simulink model "dsPIC33CK_Curiosity_CRL_ExternalMode"  (R2020b)
settings: Solver=FixedStepDiscrete  StartTime=0.0  StopTime=inf  FixedStep=0.01  RelTol=1e-3
undefined symbols (not defined in the file): B0, D3, D4, Max, MaxPer, ms, P32, P67, P68, Pin, Resol, Timer, us
libraries: MCHP_Blockset x9
(part 1 of 2)
settings Model: SimulationMode=external  ExtModeTrigDuration=1  Creator=M17129  LastModifiedBy=Lubin Kerhuel
settings DataIOCC: ReturnWorkspaceOutputs=off
settings OptimizationCC: DefaultUnderspecifiedDataType=single  EfficientTunableParamExpr=on
settings DebuggingCC: ParameterTunabilityLossMsg=error  ArithmeticOperatorsInVariantConditions=warning
settings HardwareCC: ProdBitPerInt=16  ProdBitPerPointer=16  ProdBitPerSizeT=16  ProdBitPerPtrDiffT=16  ProdLargestAtomicInteger=Integer  ProdLargestAtomicFloat=None  ProdWordSize=16  ProdHWDeviceType=Generic->Custom
settings ModelReferenceCC: ModelReferenceNumInstancesAllowed=Single
settings SFSimCC: SimUseLocalCustomCode=off  MATLABDynamicMemAlloc=off  CustomCodeUndefinedFunction=UseInterfaceOnly
settings RTWCC: Description=Microchip Embedded Target PIC24 dsPIC30 dsPIC33 (real-time)  SystemTargetFile=MCHP_dsPIC_stf.tlc  TemplateMakefile=MCHP_dsPIC.tmf  GenerateReport=on  RTWUseLocalCustomCode=off  IncludeHyperlinkInReport=on  LaunchReport=on  CodeProfilingSaveOptions=AllData  GenerateTraceInfo=on  GenerateTraceReport=on  GenerateTraceReportSl=on  GenerateTraceReportSf=on  GenerateTraceReportEml=on  GenerateWebview=on  GenerateCodeMetricsReport=on  GenerateCodeReplacementReport=on
settings CodeAppCC: ForceParamTrailComments=on  IgnoreCustomStorageClasses=off  MaxIdLength=255  OperatorAnnotations=on  SimulinkDataObjDesc=on  SFDataObjDesc=on  InsertBlockDesc=on
settings STFCustomTargetCC: TargetLibSuffix=_lib.a  CodeReplacementLibrary=Microchip Code Replacement Library for dsPIC  MultiwordLength=256  ConcurrentExecutionCompliant=off  IncludeMdlTerminateFcn=off  CombineOutputUpdateFcns=on  CombineSignalStateStructs=on  ERTCustomFileBanners=on  SupportContinuousTime=off  RemoveResetFunc=on  MATLABClassNameForMDSCustomization=Simulink.SoftwareTarget.ERTCustomization  CPPClassGenCompliant=off  GRTInterface=off  SystemTargetFile=MCHP_dsPIC_stf.tlc
settings ERTTargetCC: TargetLibSuffix=_lib.a  CodeReplacementLibrary=Microchip Code Replacement Library for dsPIC  ParMdlRefBuildCompliant=off  CompOptLevelCompliant=off  ConcurrentExecutionCompliant=off  IncludeMdlTerminateFcn=off  CombineSignalStateStructs=on  SupportNonInlinedSFcns=on  ModelStepFunctionPrototypeControlCompliant=off  CPPClassGenCompliant=off  UseToolchainInfoCompliant=off  ExtMode=on  ExtModeTransport=1  ExtModeStaticAllocSize=1024  ExtModeMexFile=ext_serial_win32_comm_no_acks  ExtModeMexArgs=1 10 460800  ERTSrcFileBannerTemplate=MCHP_dsPIC_code_template.cgt  ERTHdrFileBannerTemplate=MCHP_dsPIC_code_template.cgt  ERTDataSrcFileTemplate=MCHP_dsPIC_code_template.cgt  ERTDataHdrFileTemplate=MCHP_dsPIC_code_template.cgt  ERTCustomFileTemplate=MCHP_main.tlc

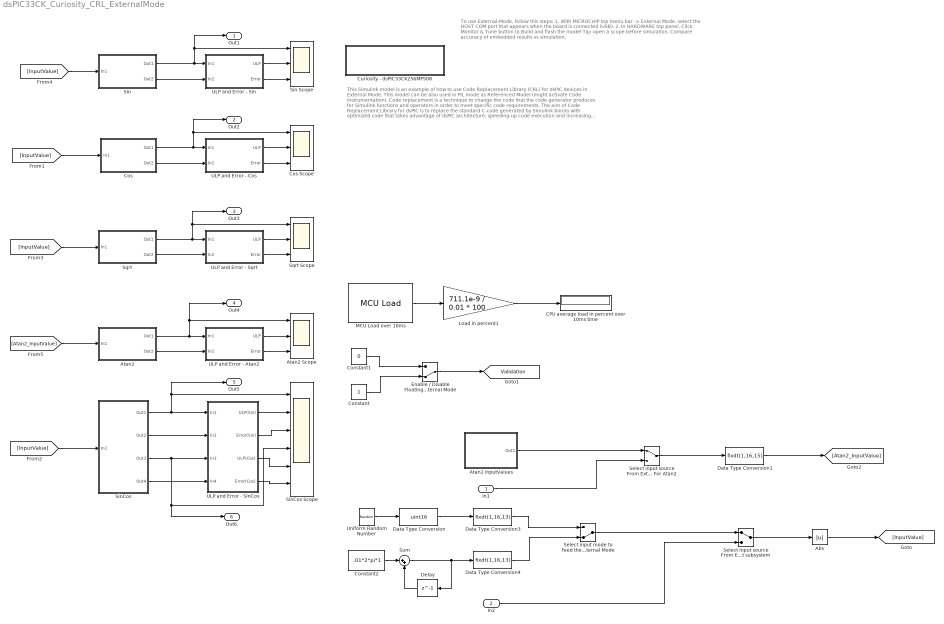
== system dsPIC33CK_Curiosity_CRL_ExternalMode ==
  note: This Simulink model is an example of how to use Code Replacement Library (CRL) for dsPIC devices in External Mode. This model can be also used in PIL mode as Referenced Model (might activate Code instrumentation).
      |
      | Code replacement is a technique to change the code that the code generator produces for Simulink functions and operators
      | in order to meet specific code requirements. The aim of Code Replacement Library for dsPIC is to replace the standard C-code generated
      | by Simulink blocks with optimized code that takes advantage of dsPIC architecture, speeding-up code execution and increasing the precision.
      |
      | Microchip Code Replacement Library for dsPIC provides support for:
      | - Fixed-Point Matrix Multiplication operations
      | - Fixed-Point Atan2
      | - Fixed-Point Sqrt and Sqrt32
      | - Fixed-Point Sin
      | - Fixed-Point Cos
      | - Fixed-Point SinCos
      | - Abs (absolute value)
      | - Addition and Subtraction with Saturation
      | - Saturation and Cast operations
      |
      | The user can enable Code Replacement Library in two easy steps:
      | 1. Open Configuration Parameters of the Simulink Model
      | 2. From Code Generation --> Interface pane select "Microchip® Code Replacement Library for dsPIC".
      |
      | *You can check which blocks triggered the code replacement by inspecting Code Replacement Report displayed at the end of the build process.
      | *Since this model runs in External Mode you can change the values of tunable parameters (ex. input values for trigonometric functions).
  note: To use External-Mode, follow this steps:
      | 1. With MICROCHIP top menu bar -> External Mode, select the HOST
      | COM port that appears when the board is connected (USB).
      | 2. In HARDWARE top panel, Click Monitor & Tune button to Build and flash the model
      |
      | Tip: open a scope before simulation.
      | Compare accuracy of embedded results vs simulation.
  In1 : Inport  PortDimensions=2
  In2 : Inport  Port=2
  Abs : Abs
  Atan2 : Subsystem
  Atan2 InputValues : Subsystem
  Atan2 Scope : Scope  NumInputPorts=3
  CPU average load in percent over 10ms time : Display
  Constant : Constant  OutDataTypeStr=uint16
  Constant1 : Constant  Value=0  OutDataTypeStr=uint16
  Constant2 : Constant  Value=.01*2*pi*1  OutDataTypeStr=fixdt(1,16,2*pi/65536,0)  SampleTime=.01
  Cos : Subsystem
  Cos Scope : Scope  NumInputPorts=3
  Curiosity - dsPIC33CK256MP508 : Subsystem
  Data Type Conversion : DataTypeConversion  OutDataTypeStr=uint16  ConvertRealWorld=Stored Integer (SI)
  Data Type Conversion1 : DataTypeConversion  OutDataTypeStr=fixdt(1,16,15)  ConvertRealWorld=Stored Integer (SI)
  Data Type Conversion3 : DataTypeConversion  OutDataTypeStr=fixdt(1,16,13)  ConvertRealWorld=Stored Integer (SI)
  Data Type Conversion4 : DataTypeConversion  OutDataTypeStr=fixdt(1,16,13)
  Delay : Delay  DelayLength=1  InitialCondition=0
  Enable / Disable Floating-Point Reference Output *Modifiable in External Mode : ManualSwitch  CurrentSetting=0
  Load in percent1 : Gain  Gain=711.1e-9 / 0.01 * 100  ParamDataTypeStr=Inherit: Inherit from 'Gain'  OutMin=[0]  OutMax=[20]  OutDataTypeStr=single
  MCU Load over 10ms : MCHP_Blockset/Profiling/MCU Load  MCULoadPin=Dynamic Options  MCULoadPin_TXT=None  MCULoadMeasure=on  TIMER_Resolution=Dynamic Options  TIMER_Resolution_TXT="Resol: 0.9143(us)  -  Max: 59.9(ms)"  MCHP_TIMER_REQUEST={MCU_Load}{MCU_Load}21:5:0:0:[]:4194304;  MCHP_TIMER_RESULT=[3 65535 ]  MCHP_MASTERLINK=dsPIC33CK_Curiosity_CRL_ExternalMode/Curiosity - dsPIC33CK256MP508/Microchip Master  MCHP_COMPILED_INFO="CompiledSampleTime= [0.010000000000000000208   0 ];CompiledInportDataTypes=[    ];CompiledInportDataWidth=[];"  Info="Timer 3:  Resol: 711.1111111(ns)  -  Max: 46.6034(ms)"  SampleTime=0.01
      settings: SourceProductName=MPLAB® Device Blocks for Simulink®
  Select input mode to feed the functions under test *Modifiable in External Mode : ManualSwitch  CurrentSetting=0
  Select input source From External (input port) / From Current subsystem : ManualSwitch
  Select input source From External (input port) / From Current subsystem For Atan2 : ManualSwitch
  Sin : Subsystem
  Sin Scope : Scope  NumInputPorts=3
  SinCos : Subsystem
  SinCos Scope : Scope  NumInputPorts=6
  Sqrt : Subsystem
  "Sqrt Scope " : Scope  NumInputPorts=3
  Sum : Sum  Inputs=|++  OutDataTypeStr=Inherit: Same as first input
  ULP and Error - Atan2 : Subsystem
  ULP and Error - Cos : Subsystem
  ULP and Error - Sin : Subsystem
  ULP and Error - SinCos : Subsystem
  ULP and Error - Sqrt : Subsystem
  Uniform Random Number : UniformRandomNumber  Minimum=0  Maximum=2^16-1  SampleTime=.01
  Out1 : Outport  VectorParamsAs1DForOutWhenUnconnected=off
  Out2 : Outport  Port=2  VectorParamsAs1DForOutWhenUnconnected=off
  Out3 : Outport  Port=3  VectorParamsAs1DForOutWhenUnconnected=off
  Out4 : Outport  Port=4  VectorParamsAs1DForOutWhenUnconnected=off
  Out5 : Outport  Port=5  VectorParamsAs1DForOutWhenUnconnected=off
  Out6 : Outport  Port=6  VectorParamsAs1DForOutWhenUnconnected=off
  tag scope: Validation=global
  wires:
  ULP and Error - Cos/2(Error) -> Cos Scope/3
  ULP and Error - Cos/1(ULP) -> Cos Scope/2
  Load in percent1/1 -> CPU average load in percent over 10ms time/1
  MCU Load over 10ms/1 -> Load in percent1/1
  ULP and Error - Sqrt/1(ULP) -> "Sqrt Scope "/2
  ULP and Error - Sqrt/2(Error) -> "Sqrt Scope "/3
  ULP and Error - Atan2/1(ULP) -> Atan2 Scope/2
  ULP and Error - Atan2/2(Error) -> Atan2 Scope/3
  Sin/1(Out1) -> Out1/1, Sin Scope/1, ULP and Error - Sin/1(In1)
  Sin/2(Out2) -> ULP and Error - Sin/2(In2)
  Cos/1(Out1) -> Cos Scope/1, Out2/1, ULP and Error - Cos/1(In1)
  Cos/2(Out2) -> ULP and Error - Cos/2(In2)
  SinCos/1(Out1) -> Out5/1, SinCos Scope/1, ULP and Error - SinCos/1(In1)
  SinCos/2(Out2) -> ULP and Error - SinCos/2(In2)
  SinCos/3(Out3) -> SinCos Scope/4, Out6/1, ULP and Error - SinCos/3(In3)
  SinCos/4(Out4) -> ULP and Error - SinCos/4(In4)
  Sqrt/1(Out1) -> "Sqrt Scope "/1, Out3/1, ULP and Error - Sqrt/1(In1)
  Sqrt/2(Out2) -> ULP and Error - Sqrt/2(In2)
  Atan2/1(Out1) -> Atan2 Scope/1, Out4/1, ULP and Error - Atan2/1(In1)
  Atan2/2(Out2) -> ULP and Error - Atan2/2(In2)
  Enable / Disable Floating-Point Reference Output *Modifiable in External Mode/1 -> [Validation]
  ULP and Error - Sin/1(ULP) -> Sin Scope/2
  ULP and Error - Sin/2(Error) -> Sin Scope/3
  Constant/1 -> Enable / Disable Floating-Point Reference Output *Modifiable in External Mode/2
  Constant1/1 -> Enable / Disable Floating-Point Reference Output *Modifiable in External Mode/1
  ULP and Error - SinCos/1(ULP(Sin)) -> SinCos Scope/2
  ULP and Error - SinCos/2(Error(Sin)) -> SinCos Scope/3
  ULP and Error - SinCos/3(ULP(Cos)) -> SinCos Scope/5
  ULP and Error - SinCos/4(Error(Cos)) -> SinCos Scope/6
  Sum/1 -> Data Type Conversion4/1, Delay/1
  Delay/1 -> Sum/2
  Constant2/1 -> Sum/1
  Data Type Conversion3/1 -> Select input mode to feed the functions under test *Modifiable in External Mode/1
  Data Type Conversion4/1 -> Select input mode to feed the functions under test *Modifiable in External Mode/2
  Data Type Conversion/1 -> Data Type Conversion3/1
  Uniform Random Number/1 -> Data Type Conversion/1
  Select input mode to feed the functions under test *Modifiable in External Mode/1 -> Select input source From External (input port) / From Current subsystem/1
  Atan2 InputValues/1(Out1) -> Select input source From External (input port) / From Current subsystem For Atan2/1
  [Atan2_InputValue] -> Atan2/1(In1)
  [InputValue] -> SinCos/1(In1)
  Select input source From External (input port) / From Current subsystem/1 -> Abs/1
  Select input source From External (input port) / From Current subsystem For Atan2/1 -> Data Type Conversion1/1
  In2/1 -> Select input source From External (input port) / From Current subsystem/2
  [InputValue] -> Sqrt/1(In1)
  [InputValue] -> Cos/1(In1)
  Data Type Conversion1/1 -> [Atan2_InputValue]
  In1/1 -> Select input source From External (input port) / From Current subsystem For Atan2/2
  Abs/1 -> [InputValue]
  [InputValue] -> Sin/1(In1)

== system dsPIC33CK_Curiosity_CRL_ExternalMode/Atan2 ==
  In1 : Inport
  Atan2 Q15 : Subsystem
  Double Atan2 - Reference : Subsystem  TreatAsAtomicUnit=on
  Out1 : Outport  VectorParamsAs1DForOutWhenUnconnected=off
  Out2 : Outport  Port=2  VectorParamsAs1DForOutWhenUnconnected=off
  wires:
  In1/1 -> Atan2 Q15/1(In1), Double Atan2 - Reference/1(In1)
  Double Atan2 - Reference/1(Simulink_Out_Q1.15) -> Out2/1
  Atan2 Q15/1(Out1) -> Out1/1
  [Validation] -> Double Atan2 - Reference/Enable

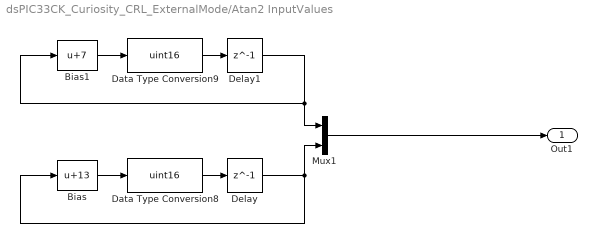
== system dsPIC33CK_Curiosity_CRL_ExternalMode/Atan2 InputValues ==
  Bias : Bias  Bias=13
  Bias1 : Bias  Bias=7
  Data Type Conversion8 : DataTypeConversion  OutDataTypeStr=uint16  ConvertRealWorld=Stored Integer (SI)
  Data Type Conversion9 : DataTypeConversion  OutDataTypeStr=uint16  ConvertRealWorld=Stored Integer (SI)
  Delay : Delay  DelayLength=1  InitialCondition=0
  Delay1 : Delay  DelayLength=1  InitialCondition=0
  Mux1 : Mux  Inputs=2
  Out1 : Outport  VectorParamsAs1DForOutWhenUnconnected=off
  wires:
  Delay/1 -> Bias/1, Mux1/2
  Data Type Conversion8/1 -> Delay/1
  Delay1/1 -> Mux1/1, Bias1/1
  Bias1/1 -> Data Type Conversion9/1
  Data Type Conversion9/1 -> Delay1/1
  Mux1/1 -> Out1/1
  Bias/1 -> Data Type Conversion8/1

== system dsPIC33CK_Curiosity_CRL_ExternalMode/Cos ==
  In1 : Inport
  Cos Double - Reference : Subsystem
  Cos Q15 : Subsystem
  Out1 : Outport  VectorParamsAs1DForOutWhenUnconnected=off
  Out2 : Outport  Port=2  VectorParamsAs1DForOutWhenUnconnected=off
  wires:
  In1/1 -> Cos Q15/1(In2), Cos Double - Reference/1(In1)
  Cos Double - Reference/1(Out1) -> Out2/1
  Cos Q15/1(Cos_Out1) -> Out1/1
  [Validation] -> Cos Double - Reference/Enable

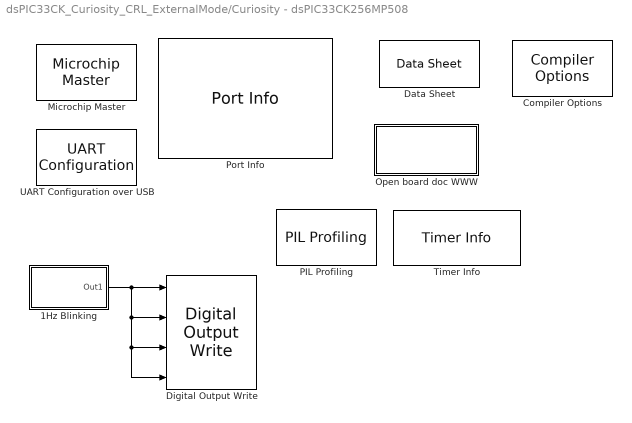
== system dsPIC33CK_Curiosity_CRL_ExternalMode/Curiosity - dsPIC33CK256MP508 ==
  1Hz Blinking : Subsystem
  Compiler Options : MCHP_Blockset/System Configuration/Compiler Options  Priority=1  LATEST_CMPLR=on  COMP_LIST=Dynamic Options  COMP_LIST_TXT=xc16 - v1.70  DFP_LIST=Dynamic Options  DFP_LIST_TXT=from compiler  CMSIS_DSP=Dynamic Options  CMSIS_DSP_TXT=Dynamic Options  USE_64BIT_DOUBLE=off  MCHP_MULTITHREAD_COMPILATION=on  UseCustom_LinkerScript=off  MCHP_MASTERLINK=dsPIC33CK_Curiosity_CRL_ExternalMode/Curiosity - dsPIC33CK256MP508/Microchip Master  OPTIMIZATION_LEVEL=2  MPLAB_LINKLIB=default  MPLAB_LINKLIB1=fast floating-point math  CodeReplacement=Dynamic Options  CodeReplacement_TXT=Microchip Code Replacement Library for dsPIC  OPTIMIZATION_FLTO=on  OPTIMIZATION_REORDER=off  UNROLL_LOOPS=off  PROCEDURAL_ABSTRACTION=off  MCODE=is less than 32768 (faster)  MCONST=in data memory  MDATA=Use only memory below address 8192 (faster)  MSCALAR=Use only memory below address 8192 (faster)  MLARGEARRAY=off  MAGGREGATE=on  HEAP_SIZE=1024  OMF=elf  DEBUG_INFO=on  ProduceHexOutput=off  AssemblyListing=off  SaveTemps=off  NO_EDS_WARN=on  PRINT_STATISTICS=off
      settings: SourceProductName=MPLAB Device Blocks for Simulink
  Data Sheet : MCHP_Blockset/System Info/Data Sheet  DOC_Type=datasheet  DOC_MCHP_Id=33CK256MP508_datasheet  DOC_FilePath=C:\Users\M91449\AppData\Local\Temp\dsPIC33CK256MP508-Family-Data-Sheet-DS70005349H.pdf  DOC_FileLastCheckTime="[2021              1             18             14             51         36.151]"  cpy_MCHP_Id=33CK256MP508  MCHP_MASTERLINK=dsPIC33CK_Curiosity_CRL_ExternalMode/Curiosity - dsPIC33CK256MP508/Microchip Master
      settings: AttributesFormatString=%<cpy_MCHP_Id>  SourceProductName=MPLAB Device Blocks for Simulink
  Digital Output Write : MCHP_Blockset/Digital IO/Digital Output Write  PORT=Dynamic Options  PORT_TXT="E   [ 0 : 15 ]"  PIN=[6 13 14 15]  PACK=off  SIMULTANEOUS=off  ORDERING=None  SampleTime=-1  MCHP_PORT={Digital Out}{DOU}1:1:E6;{Digital Out}{DOU}1:1:E13;{Digital Out}{DOU}1:1:E14;{Digital Out}{DOU}1:1:E15;  MCHP_MASTERLINK=dsPIC33CK_Curiosity_CRL_ExternalMode/Curiosity - dsPIC33CK256MP508/Microchip Master
      settings: SourceProductName=MPLAB Device Blocks for Simulink
  Microchip Master : MCHP_Blockset/System Configuration/Microchip Master  Priority=1  PICREF=33CK256MP508  TIMESTEP_REF="Timer  ( 0.01s )"  BUSYFLAG=Dynamic Options  BUSYFLAG_TXT=E5 / Pin[24]  VDD_range=Dynamic Options  PWRTEN=Not used  BOREN=Disable  BODENV=2.7V  BORV=Not used  FPWRT=128ms  DSBOREN=Enable ZPBOR during Deep Sleep Mode  DSLPBOR=Not used  MCLRE=Enabled  SMCLR=MCLR pin generates a normal system Reset  PMDL1WAY=Allow only one reconfiguration  RSTPRI=Device will obtain reset instruction from Primary flash  TEMP=Not used  SOSCSRC=Not used  SOSCSEL=Not used  IOL1WAY=Allow only one reconfiguration  ALTVREF=Not used  DISUVREG=Not used  DSSWEN=Not used  LPCFG=Not used  RTCBAT=Not used  VBTBOR=Not used  WUTSEL=Not used  POWERSAVE=off  FNOSC=Primary Oscillator (XT; HS; EC)  FPR=ECIO w/ PLL 16x  FOSFPR=HS3 w/PLL 16x  FOS=Primary Oscillator  FRANGE=High Range  OSCILLATOR_SELECT=External Clock  OSCILLATOR_SELECT_spd=External Clock  QUARTZ=8e6  QUARTZ_spd=8e6  POSCGAIN=2x gain setting  POSCBOOST=Boost the kick start of the oscillator  SOSCGAIN=2x gain setting  SOSCBOOST=Boost the kick start of the oscillator  ACTIV_PLL=on  ACTIV_PLL_spd=on  MIPS_DESIRED=90e6  MIPS_DESIRED_spd=90e6  CPUDIV=Divide by 1  FPLLMUL=Not used  FPLLIDIV=8x Divider  POSCFREQ=Not used  POSCMD=EC (External Clock) Mode  POSCMOD=Primary osc disabled  MIPS=90 * 1e6  ACLKCON=Optimized for PWM resolution & ADC conversion speed  ACLKCON_spd=Optimized for PWM resolution & ADC conversion speed  FPLLODIV=32x Divider  PLLKEN=PLL lock signal will be used to disable PLL clock output if lock is lost  FCKSM=Clock switching is enabled;Fail-safe Clock Monitor is disabled  FCKSMEN=Sw Disabled; Mon Disabled  IESO=Start up with FRC; then switch  DSWDTPS=1:2^36  FWDTEN=WDT controlled via SW; use WDTCON.ON bit  FWDTWINSZ=Window size is 25%  FWPSA=1:512  FWPSA0=1:128  FWPSB=1:16  WDT=Disable  WDTPOST=1:32768  WDTPRE=1:128  WDTPS=1:1048576  WINDIS=Watchdog Timer operates in Non-Window mode  WWDTEN=Non-Window mode  DSWDTEN=Enable DSWDT during Deep Sleep Mode  DSWDTOSC=Select LPRC as DSWDT Reference clock  FPBDIV=Not used  FSOSCEN=Disable Secondary Oscillator  LPRCSEL=Not used  OSCIOFCN=Not used  OSCIOFNC=general purpose digital I/O pin  LVRCFG=Not used  PLL_96MHZ=Not used  PLL96MHZ=Not used  PLLDIV=Not used  WDTCLK=Not used  WDTCMX=Not used  WDTWIN=WDT Window is 25% of WDT period  XTCFG=24-32 MHz crystals  XTBST=Boost the kick-start  APL=Aux Flash Code protect is disabled  APLK=Aux Flash Write Protection or Code Protection is Enabled  AWRP=Auxiliary program memory is not write-protected  BSS=No Protection (other than BWRP)  BWP=Not used  BWRP=Boot Segment may be written  CP=Protection Disabled  EBS=No Boot EEPROM  ESS=No Segment Data EEPROM  GCP=General Segment Code protect is Disabled  GSS=No Protection (other than GWRP)  GSS0=Not used  GSSK=General Segment Write Protection or Code Protection is Enabled  GWRP=General Segment may be written  PWP=Not used  RBS=No Boot RAM  RSS=No Secure RAM  SSS=No Secure Segment  SWRP=Secure segment may be written  WPCFG=Not used  WPDIS=Not used  WPEND=Not used  WPFP=Not used  ICESEL=Communicate on PGEC1/PGED1  ICS=Communicate on PGC3 and PGD3  JTAGEN=Disable  COE=Not used  RES=Not used  DEBUG=Debugger is disabled  BACKBUG=Not used  BKBUG=Not used  ALTI2C=I2C mapped to SDA1/SCL1 pins  ALTI2C1=I2C1 mapped to SDA1/SCL1 pins  ALTI2C2=I2C2 mapped to SDA2/SCL2 pins  ALTI2C3=I2C3 mapped to SDA3/SCL3 pins  ALTQIO=QEA1; QEB1; INDX1 are selected as inputs to QEI1  ALTSS1=SS1A is selected as the I/O pin for SPI1  CMPPOL0=Hysteresis is applied to falling edge  CMPPOL1=Hysteresis is applied to falling edge  FCANIO=Not used  FETHIO=Default Ethernet I/O  FMIIEN=MII Enabled  FSRSSEL=Not used  FUSBIDIO=Controlled by the USB Module  FVBUSONIO=Not used  HPOL=PWM module high side output pins have active-high output polarity  HYST0=45 mV Hysteresis  HYST1=45 mV Hysteresis  I2C1SEL=Not used  LPOL=PWM module low side output pins have active-high output polarity  PWMPIN=PWM module pins controlled by PORT register at device Reset  RTCOSC=Not used  UPLLEN=USB PLL Disabled  UPLLIDIV=Not used  ATMOD8=Not used  ALTPMP=Not used  I2C2SEL=Not used  ALTADREF=Not used  ALTCVREF=Not used  PWMLOCK=PWM registers may be written without key sequence  INT_PRIORITY_DMA=0  MCHP_TIMER_REQUEST={Time Step}{TS}0:2:3:1:[]:900000;  MCHP_TIMER_RESULT=[2 56249.000000000014552 ]  MCHP_PORT={Busy Flag}{Busy}0:1:E5;  MCHP_PLLRegisters="[1    135  16386     -1     49]"  MCHPVAR=MCHP.fcy.MIPS=90000000;MCHP.fcy.SYSCLK=90000000;MCHP.fcy.ADC=90000000;MCHP.fcy.Comparator=90000000;MCHP.fcy.I2C=90000000;MCHP.fcy.SPI=90000000;MCHP.fcy.UART=1.8e+08;MCHP.fcy.Timers=90000000;MCHP.fcy.OC=90000000;MCHP.fcy.IC=90000000;MCHP.fcy.Ports=90000000;MCHP.fcy.QEI=90000000;MCHP.fcy.APLL=-1;MCHP.PowerSave=0;MCHP.TimeStepFactor=MCHP_Fun.Hex2num('3FEFFFFFFFFFFFFE');MCHP.TimeStep_Timer=2;MCHP.NTIMERS=1;MCHP.id.name='33CK256MP508';MCHP.id.N=reshape([33 256 508],1,3);MCHP.id.L=reshape({ 'CK','MP',''},1,3);MCHP.id.Arch=3;MCHP.periph.PPS.reg_RPINRx=reshape([-1 1 1 1 -1 1 1 1 1 1 1 1 1 1 1 1 1 1 1 1 1 1 -1 -1 1 1 1 1 1 1 1 1 1 1 1 1 1 1 1 1 1 1 1 -1 1 1 1 -1 -1 -1 -1 -1 1 -1 1 1 -1 -1 1 1 1 -1 -1 -1 -1 1 1 -1 -1 -1 -1 -1 -1 -1 -1 1 1 -1 -1 -1 -1 -1 -1 -1 1 1 1 1 1 1 1 -1 -1 -1 -1 -1 -1 1 1 1],1,100);MCHP.PPS.dsPIC.RP=reshape([-1 -1 -1 -1 -1 -1 -1 -1 -1 -1 -1 -1 -1 -1 -1 -1 -1 -1 -1 -1 -1 -1 -1 -1 -1 -1 -1 -1 -1 -1 -1 -1 16 17 18 19 20 21 22 23 24 25 26 27 28 29 30 31 32 32 33 35 36 37 38 34 40 41 42 43 44 45 46 47 48 49 50 51 52 53 54 55 56 57 35 59 60 61 62 63],1,80);MCHP.PPS.dsPIC.RPI=reshape(MCHP_Fun.Hex2num('[]'),0,0);MCHP.PPS.dsPIC.RPINR_list=reshape({ '1','INT1','INT2','INT3','5','T1CK','TCKI1','ICM1','TCKI2','ICM2','TCKI3','ICM3','TCKI4','ICM4','TCKI5','ICM5','TCKI6','ICM6','TCKI7','ICM7','TCKI8','ICM8','OCFA','OCFB','PCI8','PCI9','PCI10','PCI11','QEIA1','QEIB1','QEINDX1','QEIHOM1','QEIA2','QEIB2','QEINDX2','QEIHOM2','U1RX','U1DSR','U2RX','U2DSR','SDI1','SCK1_in','SS1_in','REFOI','SDI2','SCK2_in','SS2_in','48','49','50','51','52','CAN1RX','54','U3RX','U3DSR','57','58','SDI3','SCK3_in','SS3_in','62','63','64','65','TCKI9','ICM9','68','69','70','71','72','73','74','OCFC','PCI17','PCI18','78','79','80','81','82','83','84','PCI12','PCI13','PCI14','PCI15','PCI16','SENT1','SENT2','CLCINA','CLCINB','CLCINC','CLCIND','ADCTRG','OCFD','U1CTS','U2CTS','U3CTS'},1,100);MCHP.PPS.dsPIC.RPOR_list=reshape({ '1','U1TX','U1RTS','U2TX','U2RTS','SDO1','SCK1_out','SS1_out','SDO2','SCK2_out','SS2_out','SDO3','SCK3_out','SS3_out','REFCLKO','OCM1','OCM2','OCM3','OCM4','OCM5','OCM6','CAN1','22','CMP1','CMP2','CMP3','26','U3TX','U3RTS','29','30','31','32','33','PWM4H','PWM4L','PWMEA','PWMEB','QEICCMP1','QEICCMP2','CLC1OUT','CLC2OUT','OCM7','OCM8','PWMEC','PWMED','PTGTRG24','PTGTRG25','SENT1OUT','SENT2OUT','MCCP9A','MCCP9B','MCCP9C','MCCP9D','MCCP9E','MCCP9F','56','57','58','CLC3OUT','CLC4OUT','U1DTR','U2DTR','U3DTR'},1,64);MCHP.PPS.map_RPnR_RPORx=reshape([32 33 34 35 36 37 38 39 40 41 42 43 44 45 46 47 48 49 50 51 52 53 54 55 56 57 58 59 60 61 62 63 64 65 66 67 68 69 70 71 72 73 74 75 76 77 78 79 176 177 178 179 180 181],1,54);MCHP.Rx=reshape([16 34 15 74 2 -1 -1 -1 -1 -1 -1 18 35 28 73 4 -1 -1 -1 -1 -1 -1 20 41 29 72 17 -1 -1 -1 -1 -1 -1 21 43 33 69 19 -1 -1 -1 -1 -1 -1 23 45 63 68 22 -1 -1 -1 -1 -1 -1 -1 55 65 54 24 -1 -1 -1 -1 -1 -1 -1 56 30 53 37 -1 -1 -1 -1 -1 -1 -1 58 40 52 39 -1 -1 -1 -1 -1 -1 -1 60 46 49 42 -1 -1 -1 -1 -1 -1 -1 61 47 48 44 -1 -1 -1 -1 -1 -1 -1 75 66 38 57 -1 -1 -1 -1 -1 -1 -1 76 67 36 59 -1 -1 -1 -1 -1 -1 -1 78 5 27 62 -1 -1 -1 -1 -1 -1 -1 80 6 14 64 -1 -1 -1 -1 -1 -1 -1 1 7 13 77 -1 -1 -1 -1 -1 -1 -1 3 8 10 79 -1 -1 -1 -1 -1 -1],11,16);MCHP.ADC.ANtype=reshape([0 0],1,2);MCHP.ADC.ADCONx=reshape([0 0 0 0 0 0],1,6);MCHP.ADC.ADCHS_0=reshape([0 0],1,2);MCHP.ADC.Flags=reshape([-1 0],1,2);MCHP.ADC.Buffer=reshape([-1 -1],1,2);MCHP.ADC.port=reshape([0 18 23 3 4 16 17 -1 19 2 24 25 32 33 34 35 39 38 58 59 64 65 66 67 -1 -1 -1 -1 -1 -1 -1 -1 -1 -1 -1 -1 -1 -1 -1 -1 -1 -1 -1 -1 -1 -1 -1 -1 -1 -1 -1 -1 -1 -1 -1 -1 -1],1,57);MCHP.ADC.port_ALT=reshape([18 1 -1 -1],1,4);MCHP.ADC.port_VrefP=-1;MCHP.ADC.port_VrefM=-1;MCHP.ADC.port_AVdd=-1;MCHP.ADC.port_AVss=-1;MCHP.ADC.ADCDATA=reshape([1 1 1 1 1 1 1 1 1 1 1 1 1 1 1 1 1 1 1 1 1 1 1 1 1 1 0 0 0 0 0 0 0 0 0 0 0 0 0 0 0 0 0 0 0 0 0 0 0 0 0 0 0 0 0 0 0],1,57);MCHP.ADC.HS_SAR.TRGSRC=reshape([1 1 1 1 1 1 1 1 1 1 1 1 1 1 1 1 1 1 1 1 1 1 1 1 1 1],1,26);MCHP.ADC.HS_SAR.nFilters=4;MCHP.ADC.HS_SAR.nDedicatedCore=2;MCHP.ADC.HS_SAR.CALIBRATION=0;MCHP.ADC.HS_SAR.ADCON1L=40960;MCHP.ADC.HS_SAR.ADC_Class3_idxStart=26;MCHP.memory.RAM=24576;MCHP.memory.RAM_XBegin=4096;MCHP.memory.RAM_YBegin=20480;MCHP.memory.RAM_dma=reshape([-1 -1],1,2);MCHP.memory.FLASH_ECC=0;MCHP.DMA.Num=0;MCHP.DMA.CNTmax=0;MCHP.QEI.QEICONx=reshape([49023 49023 -1 -1 -1 -1],1,6);MCHP.QEI.QEItype=2;MCHP.QEI.Port_QEI_INDX=reshape([-1 -1],1,2);MCHP.QEI.Port_QEI_QEA=reshape([-1 -1],1,2);MCHP.QEI.Port_QEI_QEB=reshape([-1 -1],1,2);MCHP.QEI.Port_QEI_UPDN=reshape([-1 -1],1,2);MCHP.INT.Port=reshape([18 32767 32767 32767 -1],1,5);MCHP.PWM_HS.Flags=reshape([0 0 0],1,3);MCHP.PWM.port_FLT=reshape([-1 -1 -1 -1 -1 -1 -1 -1 -1 -1 -1 -1 -1 -1 -1 -1 -1 -1 -1 -1 -1 -1 -1 -1 -1 -1 -1 -1 -1 -1 -1 -1 -1],1,33);MCHP.PWM.PWMRef=-1;MCHP.PWM.Flag=0;MCHP.PWM.Port_PWM_l=reshape([31 -1 29 -1 27 -1 48 -1 37 -1 47 -1 43 -1 45 -1 -1 -1 -1 -1 -1 -1 -1 -1],2,12);MCHP.PWM.Port_PWM_h=reshape([30 -1 28 -1 26 -1 49 -1 36 -1 46 -1 42 -1 44 -1 -1 -1 -1 -1 -1 -1 -1 -1],2,12);MCHP.PWM_HS_FEP.nEVTOUT=5;MCHP.IC.Port=reshape([0 0 0 0 0 0 0 0 0 0 0 0 0 0 0 0],1,16);MCHP.IC.type=-1;MCHP.OC.Port=reshape([0 0 0 0 0 0 0 0 0 0 0 0 0 0 0 0],1,16);MCHP.OC.type=-1;MCHP.CN.Port=reshape([-1 -1 -1 -1 -1 -1 -1 -1 -1 -1 -1 -1 -1 -1 -1 -1 -1 -1 -1 -1 -1 -1 -1 -1 -1 -1 -1 -1 -1 -1 -1 -1 -1 -1 -1 -1 -1 -1 -1 -1 -1 -1 -1 -1 -1 -1 -1 -1 -1 -1 -1 -1 -1 -1 -1 -1 -1 -1 -1 -1 -1 -1 -1 -1 -1 -1 -1 -1 -1 -1 -1 -1 -1 -1 -1 -1 -1 -1 -1 -1 -1 -1 -1 -1 -1],1,85);MCHP.CN.PullUp=reshape([31 65535 65535 65535 65535 0 0 0 0 0 0],1,11);MCHP.CN.type=1;MCHP.CN.Flag_PullDown=1;MCHP.SPI.Refs=reshape([1 2 3 0 0 0],1,6);MCHP.SPI.SPIxCON1=-1;MCHP.SPI.SPIxCON2=-1;MCHP.SPI.Port_SDI=reshape([-1 41 -1 -1 -1 -1],1,6);MCHP.SPI.Port_SDO=reshape([-1 56 -1 -1 -1 -1],1,6);MCHP.SPI.Port_SCK=reshape([-1 40 -1 -1 -1 -1],1,6);MCHP.SPI.Port_SS=reshape([-1 -1 -1 -1 -1 -1],1,6);MCHP.I2C.Refs=reshape([1 2 3 0 0],1,5);MCHP.I2C.I2CxCON=49151;MCHP.I2C.NewRegName=2;MCHP.I2C.Port_SDA=reshape([25 21 23 -1 -1],1,5);MCHP.I2C.Port_SCL=reshape([24 22 18 -1 -1],1,5);MCHP.I2C.Port_ASDA=reshape([40 36 52 -1 -1],1,5);MCHP.I2C.Port_ASCL=reshape([41 37 51 -1 -1],1,5);MCHP.I2C.Fuse_Port_SCL_SDA=reshape([28 1 29 1 30 1 -1 -1 -1 -1],2,5);MCHP.I2C.Fuse_Port_ASCL_ASDA=reshape([28 2 29 2 30 2 -1 -1 -1 -1],2,5);MCHP.SCCP.nSCCP=9;MCHP.SCCP.MCCP=reshape([0 0 0 0 0 0 0 0 1],1,9);MCHP.PGA.Port_PGA1P=reshape([-1 -1 -1 -1],1,4);MCHP.PGA.Port_PGA1N=reshape([-1 -1 -1 -1],1,4);MCHP.PGA.Port_PGA2P=reshape([-1 -1 -1 -1],1,4);MCHP.PGA.Port_PGA2N=reshape([-1 -1 -1 -1],1,4);MCHP.PGA.Num=0;MCHP.HS_AnalogComparator.Port_CMP1=reshape([0 33 3 18],1,4);MCHP.HS_AnalogComparator.Port_CMP2=reshape([35 34 59 18],1,4);MCHP.HS_AnalogComparator.Port_CMP3=reshape([23 4 58 18],1,4);MCHP.HS_AnalogComparator.Port_CMP4=reshape([-1 -1 -1 -1],1,4);MCHP.HS_AnalogComparator.PORT_EXTREFx=reshape([-1 -1],1,2);MCHP.HS_AnalogComparator.Port_DACOUTx=reshape([3 -1],1,2);MCHP.HS_AnalogComparator.Num=0;MCHP.Comp.Port_CVrefin=-1;MCHP.Comp.Port_CVref=-1;MCHP.Comp.Port_CVref1O=-1;MCHP.Comp.Port_CVref2O=-1;MCHP.Comp.Port_CxOUT=reshape([32767 32767 32767 32767 32767],1,5);MCHP.Comp.Port_OAxOUT=reshape([0 18 4 -1 -1],1,5);MCHP.Comp.Port_CxINP=reshape([-1 -1 -1 -1 -1],1,5);MCHP.Comp.Port_CxINM=reshape([-1 -1 -1 -1 -1 -1 -1 -1 -1 -1 -1 -1 -1 -1 -1 -1 -1 -1 -1 -1],4,5);MCHP.Comp.Port_OAxINP=reshape([2 20 34 -1 -1],1,5);MCHP.Comp.Port_OAxINM=reshape([1 19 33 -1 -1],1,5);MCHP.Comp.nComp=reshape([5 0 0],1,3);MCHP.Comp.OpAmp=0;MCHP.Comp.CVRCON=reshape([0 0],1,2);MCHP.Comp.CMCON=0;MCHP.CDAC.Port_DACx=reshape([-1 -1 -1],1,3);MCHP.CDAC.nCDAC=0;MCHP.UART.port_Rx=reshape([32767 32767 32767 -1 -1 -1],1,6);MCHP.UART.port_Tx=reshape([32767 32767 32767 -1 -1 -1],1,6);MCHP.UART.port_ARx=reshape([-1 -1],1,2);MCHP.UART.port_ATx=reshape([-1 -1],1,2);MCHP.UART.port_RTS=reshape([32767 32767 32767 -1 -1 -1],1,6);MCHP.UART.port_CTS=reshape([32767 32767 32767 -1 -1 -1],1,6);MCHP.UART.reg_UxMODE=reshape([48127 48127 48127 -1 -1 -1],1,6);MCHP.UART.reg_UxSTA=reshape([65535 65535 65535 -1 -1 -1],1,6);MCHP.modsrc.DOS_02551_cpu_16bit_v7=1;MCHP.modsrc.DOS_01520_wdt_dmt_upb_v1_16bit=1;MCHP.modsrc.DOS_02359a_sent_j2716_upb_v1=1;MCHP.modsrc.DOS_02672_math_progcrc_upb_v1_16bit=1;MCHP.modsrc.DOS_01577_cla_clc_upb_v1=1;MCHP.modsrc.DOS_02915_ecc_v2=1;MCHP.modsrc.DOS_02673_tmr_classa_upb_v1_16bit=1;MCHP.modsrc.DOS_01494_qei_32b_upb_v1_16bit=1;MCHP.modsrc.DOS_02552_msi_upb_v1_Master=0;MCHP.modsrc.DOS_01441_i2c_upb_v1_16bit_TLAH=1;MCHP.modsrc.DOS_03076_uart_protocol_upb_v1_16bit=1;MCHP.modsrc.DOS_01482=1;MCHP.modsrc.DOS_01483_pwm_16bit=1;MCHP.modsrc.DOS_02497_WACV=0;MCHP.modsrc.DOS_02316_nvm_ctrl_v1_16bit=1;MCHP.modsrc.DOS_02653_afe_current_bias_ctrl_upb_v1_16bit=1;MCHP.modsrc.DOS_01459_ptg_pc_upb_v1_16bit=1;MCHP.modsrc.DOS_01512_ccp_mccp_upb_v1_16bit=1;MCHP.modsrc.DOS_02519_dma_sfr_16bit_v2=1;MCHP.modsrc.DOS_02508c11=1;MCHP.modsrc.DOS_02475_dac_pdm_nbit_upb_v1_16bit=1;MCHP.modsrc.DOS_02467_gpio_upb_v1_16bit=1;MCHP.modsrc.DOS_00805_rst_integration_v4=1;MCHP.modsrc.DOS_02659_clk_sib_v12=1;MCHP.modsrc.DOS_02674_wdt_upb_v1_16bit=1;MCHP.modsrc.DOS_01407=1;MCHP.modsrc.DOS_02552_msi_upb_v1_Slave=0;MCHP.modsrc.DOS_02593_amp_pga_ctrl_pb_v2_16bit=0;MCHP.modsrc.DOS_03247_CAN_FD_UPB_V2_16_bit=1;MCHP.modsrc.DOS_01461_afe_ctmu_con_upb_v1_16bit=0;MCHP.modsrc.DOS_02497_WACA=0;MCHP.modsrc.DOS_02478_uart_irda_upb_v1_16bit=0;MCHP.modsrc.DOS_00929=0;MCHP.modsrc.DOS_01198=0;MCHP.modsrc.DOS_03029_WACH=0;MCHP.modsrc.DOS_02949_WACG=1;MCHP.modsrc.DOS_03349_amp_pad_opamp_ctrl_upb_v1=1;MCHP.modsrc.DOS_02237_osc_dco_ctrl_upb_v1_16bit=1;MCHP.modsrc.DOS_02472_ppi_pmp16_upb_v1_16bit=1;MCHP.modsrc.DOS_03994_WAC07=0;MCHP.modsrc.DOS_03662_WACU=0;MCHP.modsrc.DOS_00794=0;MCHP.modsrc.DOS_00931=0;MCHP.modsrc.DOS_00932=0;MCHP.modsrc.DOS_00942=0;MCHP.modsrc.DOS_00938=0;MCHP.modsrc.DOS_00996=0;MCHP.modsrc.DOS_00997=0;MCHP.modsrc.DOS_00998=0;MCHP.modsrc.DOS_00209=0;MCHP.modsrc.DOS_01555_adc=0;MCHP.modsrc.DOS_01293=0;MCHP.modsrc.DOS_00828=0;MCHP.modsrc.DOS_01116=0;MCHP.modsrc.DOS_01017_RPORx=0;MCHP.modsrc.DOS_01017_RPINRx=0;MCHP.modsrc.DOS_01555_nvm_tsmc18_v2_16bit=0;MCHP.modsrc.DOS_00804=0;MCHP.modsrc.DOS_00826=0;MCHP.modsrc.DOS_01555_TLAK_PMDx=0;MCHP.modsrc.DOS_01555_TLAK_INT_=0;MCHP.modsrc.DOS_00933=0;MCHP.modsrc.DOS_01555=0;MCHP.modsrc.DOS_01555_ptg=0;MCHP.modsrc.DOS_00958=0;MCHP.modsrc.DOS_01117_PORTx=0;MCHP.modsrc.DOS_00999=0;MCHP.modsrc.DOS_01041=0;MCHP.modsrc.DOS_00892=0;MCHP.modsrc.DOS_01287_TLAC_PMDx=0;MCHP.modsrc.DOS_01287_TLAC_INT_=0;MCHP.modsrc.DOS_01424=0;MCHP.modsrc.DOS_01332=0;MCHP.modsrc.DOS_01468_PMBA_current_source=0;MCHP.modsrc.DOS_02291_PGA=0;MCHP.modsrc.DOS_01467_Comparator=0;MCHP.modsrc.DOS_01498_TLAY=0;MCHP.modsrc.DOS_00993_PLL_120MHz=0;MCHP.modsrc.DOS_01332_ptg_pc_v1=0;MCHP.modsrc.DOS_00958_pwm_TLAY=0;MCHP.modsrc.TLAY_IOPorts=0;MCHP.modsrc.DOS_00929q=0;MCHP.modsrc.DOS_02415_spi_v5=0;MCHP.modsrc.DOS_RPINRx_16bit_2=0;MCHP.modsrc.DOS_01497_TLAH_PMDx=0;MCHP.modsrc.DOS_02550_TLAL_INT=0;MCHP.modsrc.DOS_00958_pwm_TLAH=0;MCHP.modsrc.DOS_01287_TLAH_INT_=0;MCHP.modsrc.DOS_01113=0;MCHP.modsrc.DOS_01017_PMDx=0;MCHP.modsrc.DOS_00927=0;MCHP.modsrc.DOS_01080=0;MCHP.modsrc.DOS_00794_cpu_16bit_v3=0;MCHP.modsrc.DOS_02192_TLCD_PMDx=0;MCHP.modsrc.DOS_02192_TLCD_INT_=0;MCHP.modsrc.DOS_02192_cmp=0;MCHP.modsrc.DOS_00958_pwm_TLCD=0;MCHP.modsrc.DOS_02192_PORTx_TLCD=0;MCHP.modsrc.DOS_00936=0;MCHP.modsrc.DOS_00995=0;MCHP.modsrc.DOS_00546=0;MCHP.modsrc.DOS_00474=0;MCHP.modsrc.DOS_02481_WACK_MC_Config=0;MCHP.modsrc.DOS_03088_pfm_cache_ocp_v2_WACK=0;MCHP.modsrc.DOS_02819_pfm_ctrl_32bit_upb_v2=0;MCHP.modsrc.DOS_02674_wdt_upb_v1_32bit=0;MCHP.modsrc.DOS_01520_wdt_dmt_upb_v1=0;MCHP.modsrc.DOS_02869_icd_jtag_bvci_upb_v2=0;MCHP.modsrc.DOS_02823_WACJ_clk_cru_upb_v2=0;MCHP.modsrc.DOS_02823_WACN_clk_cru_upb_v2=0;MCHP.modsrc.DOS_01423_RPINRx=0;MCHP.modsrc.DOS_02481_RPORx=0;MCHP.modsrc.DOS_02511_pwr_sib_upb_v1_32bit=0;MCHP.modsrc.DOS_02907_WACN_GP_int_evic_v3=0;MCHP.modsrc.DOS_01500_dma_bvci_v2=0;MCHP.modsrc.DOS_02141_tmr_classa_pb_v2=0;MCHP.modsrc.DOS_02815_tmr_classb_upb_v1=0;MCHP.modsrc.DOS_00740_icap_pb_v1=0;MCHP.modsrc.DOS_00749_ocmp_pb_v1=0;MCHP.modsrc.DOS_01441_i2c_upb_v1_32bit=0;MCHP.modsrc.DOS_01329_spi_pb_v2=0;MCHP.modsrc.DOS_02478_uart_irda_upb_v1_32bit=0;MCHP.modsrc.DOS_03554_cmp_control_upb_v2_32bit=0;MCHP.modsrc.DOS_01445_dac_nbit__control_upb_v1_32bit=0;MCHP.modsrc.DOS_01461_afe_ctmu_con_upb_v1=0;MCHP.modsrc.DOS_01577_cla_clc_upb_v1_32bit=0;MCHP.modsrc.DOS_02467_gpio_ports_upb_v1=0;MCHP.modsrc.DOS_02508_adc_sar_ctrl_upb_v1_PIC32MK=0;MCHP.modsrc.DOS_01261_tmr_rtcc_pb_v2=0;MCHP.modsrc.DOS_01475_lpwr_deep_sleep_ctrl_v2=0;MCHP.modsrc.DOS_EIP_00136_ssx_v1=0;MCHP.modsrc.DOS_02907_WACN_MC_int_evic_v3=0;MCHP.modsrc.DOS_01477_pwm_mc_upb_v1=0;MCHP.modsrc.DOS_01494_qei_32b_upb_v1=0;MCHP.modsrc.DOS_03247_can_fd_upb_v2_pic32mk=0;MCHP.modsrc.DOS_02907_WACK_MC_int_evic_v3=0;MCHP.modsrc.DOS_02514_dfm_strl_sst_upb_v1=0;MCHP.modsrc.DOS_02472_ppi_pmp16_upb_v1=0;MCHP.modsrc.DOS_02813a_usb_otgcore_pb_v3=0;MCHP.modsrc.DOS_02481_WACJ_MC_Config=0;MCHP.modsrc.DOS_02569_pfm_cache_ocp_v1=0;MCHP.modsrc.DOS_02481_WACJ_MC_int_evic_v3=0;MCHP.modsrc.DOS_01459_ptg_pc_upb_v1_SIC=0;MCHP.modsrc.DOS_01427_cmp_control_upb_v1_32bit=0;MCHP.modsrc.DOS_01152_can_bvci_v1=0;MCHP.modsrc.DOS_02787_WACD_Config=0;MCHP.modsrc.DOS_00800_dac_4bit_ctrl_pb_v1=0;MCHP.modsrc.DOS_01539_icd_jtag_pb_v2=0;MCHP.modsrc.DOS_02823_clk_cru_upb_v2=0;MCHP.modsrc.DOS_01423_RPORx=0;MCHP.modsrc.DOS_02907_WACD_int_evic_v3=0;MCHP.modsrc.DOS_00734_uart_irda_pb_v1=0;MCHP.modsrc.DOS_00687_tmr_classa_pb_v1=0;MCHP.modsrc.DOS_00745_tmr_classb_pb_v1=0;MCHP.modsrc.DOS_02508_adc_sar_ctrl_upb_v1=0;MCHP.modsrc.DOS_00866_cmp_control_pb_v2=0;MCHP.modsrc.DOS_01114_eth_bvci_v1=0;MCHP.modsrc.DOS_02831_usb_clk_rst_v2=0;MCHP.modsrc.DOS_01643_pfm_cache_ahb_v2=0;MCHP.modsrc.DOS_EIP_00206r5_sqi_v2=0;MCHP.modsrc.DOS_EIP_00124_usb_hs_otgcore_v1=0;MCHP.modsrc.DOS_EIP_00218_math_rng_ahbs_v2=0;MCHP.modsrc.DOS_EIP_00109_ebi_v1=0;MCHP.modsrc.DOS_EIP_00158_crypto_v1=0;MCHP.PortBase=16;MCHP.PortPrefixe='P';MCHP.clock.PBxDIV=-1;  MCHP_CRC=15922927  BTMODE=Not used  RES1=Not used  PLLSS=Not used  RES2=Not used  ALTCMPI=Not used  BOREN1=Not used  ALTRB6=Not used  RETCFG=Not used  DFMCY=Not used  BSS2=No Boot Segment  BSEN=No Boot Segment  CWRP=Configuration Segment may be written  CSS=No Protection (other than CWRP)  AIVTDIS=Disabled AIVT  BSLIM=Not used  WDTEN=Disable  BTSWP=BOOTSWP instruction is disabled  DBCC=No Cross Connection between DAC outputs  CTXT1=Not Assigned  CTXT2=Not Assigned  SEQNUM=Not used  nSEQNUM=Not used  BOREN0=Enabled  DMTIVT=Not used  DMTCNT=2^8 (256)  DMTEN=Dead Man Timer is Disabled and can be enabled by software  ON=Not used  USERID=Not used  RESERVED1=Not used  PGL1WAY=Allow only one reconfiguration  FPLLRNG=34-68 MHz Input  FPLLICLK=FRC is input to the System PLL  FPLLMULT=PLL Multiply by 128  UPLLFSEL=USB PLL input is 24 MHz  DMTINTV=Window/Interval value is 127/128 counter value  WDTSPGM=WDT stops during Flash programming  FDMTEN=Deadman Timer is disabled  TRCEN=Trace features in the CPU are enabled  BOOTISA=Boot code and Exception code is MIPS32  FECCCON=ECC and Dynamic ECC are disabled (ECCCON bits are writable)  EXTDDRSIZE=Not used  FSLEEP=Flash is powered down when the device is in Sleep mode  DBGPER=Allow CPU access to all permission regions  EJTAGBEN=Normal EJTAG functionality  TSEQ=Not used  CSEQ=Not used  RWDTPS=1:1024  RCLKSEL=Always use LPRC  SWDTPS=1:1024  DMTIVTL=Not used  DMTIVTH=Not used  DMTCNTL=Not used  DMTCNTH=Not used  DMTDIS=Dead Man Timer is Disabled and can be enabled by software  SMBEN=SMBus input threshold is enabled  SPI2PIN=SPI2 uses I/O remap (PPS) pins  CTXT3=Not Assigned  CTXT4=Not Assigned  MBXM0=Mailbox register configured for Master data read (Slave to Master data transfer)  MBXM1=Mailbox register configured for Master data read (Slave to Master data transfer)  MBXM2=Mailbox register configured for Master data read (Slave to Master data transfer)  MBXM3=Mailbox register configured for Master data read (Slave to Master data transfer)  MBXM4=Mailbox register configured for Master data read (Slave to Master data transfer)  MBXM5=Mailbox register configured for Master data read (Slave to Master data transfer)  MBXM6=Mailbox register configured for Master data read (Slave to Master data transfer)  MBXM7=Mailbox register configured for Master data read (Slave to Master data transfer)  MBXM8=Mailbox register configured for Master data read (Slave to Master data transfer)  MBXM9=Mailbox register configured for Master data read (Slave to Master data transfer)  MBXM10=Mailbox register configured for Master data read (Slave to Master data transfer)  MBXM11=Mailbox register configured for Master data read (Slave to Master data transfer)  MBXM12=Mailbox register configured for Master data read (Slave to Master data transfer)  MBXM13=Mailbox register configured for Master data read (Slave to Master data transfer)  MBXM14=Mailbox register configured for Master data read (Slave to Master data transfer)  MBXM15=Mailbox register configured for Master data read (Slave to Master data transfer)  MBXHSA=MSIxMBXD15 assigned to mailbox handshake protocol block A  MBXHSB=MSIxMBXD15 assigned to mailbox handshake protocol block B  MBXHSC=MSIxMBXD15 assigned to mailbox handshake protocol block C  MBXHSD=MSIxMBXD15 assigned to mailbox handshake protocol block D  MBXHSE=MSIxMBXD15 assigned to mailbox handshake protocol block E  MBXHSF=MSIxMBXD15 assigned to mailbox handshake protocol block F  MBXHSG=MSIxMBXD15 assigned to mailbox handshake protocol block G  MBXHSH=MSIxMBXD15 assigned to mailbox handshake protocol block H  HSAEN=Mailbox data flow control handshake protocol block disabled  HSBEN=Mailbox data flow control handshake protocol block disabled  HSCEN=Mailbox data flow control handshake protocol block disabled  HSDEN=Mailbox data flow control handshake protocol block disabled  HSEEN=Mailbox data flow control handshake protocol block disabled  HSFEN=Mailbox data flow control handshake protocol block disabled  HSGEN=Mailbox data flow control handshake protocol block disabled  HSHEN=Mailbox data flow control handshake protocol block disabled  CPRA0=Master core owns pin  CPRA1=Master core owns pin  CPRA2=Master core owns pin  CPRA3=Master core owns pin  CPRA4=Master core owns pin  CPRB0=Master core owns pin  CPRB1=Master core owns pin  CPRB2=Master core owns pin  CPRB3=Master core owns pin  CPRB4=Master core owns pin  CPRB5=Master core owns pin  CPRB6=Master core owns pin  CPRB7=Master core owns pin  CPRB8=Master core owns pin  CPRB9=Master core owns pin  CPRB10=Master core owns pin  CPRB11=Master core owns pin  CPRB12=Master core owns pin  CPRB13=Master core owns pin  CPRB14=Master core owns pin  CPRB15=Master core owns pin  CPRC0=Master core owns pin  CPRC1=Master core owns pin  CPRC2=Master core owns pin  CPRC3=Master core owns pin  CPRC4=Master core owns pin  CPRC5=Master core owns pin  CPRC6=Master core owns pin  CPRC7=Master core owns pin  CPRC8=Master core owns pin  CPRC9=Master core owns pin  CPRC10=Master core owns pin  CPRC11=Master core owns pin  CPRC12=Master core owns pin  CPRC13=Master core owns pin  CPRC14=Master core owns pin  CPRC15=Master core owns pin  CPRD0=Master core owns pin  CPRD1=Master core owns pin  CPRD2=Master core owns pin  CPRD3=Master core owns pin  CPRD4=Master core owns pin  CPRD5=Master core owns pin  CPRD6=Master core owns pin  CPRD7=Master core owns pin  CPRD8=Master core owns pin  CPRD9=Master core owns pin  CPRD10=Master core owns pin  CPRD11=Master core owns pin  CPRD12=Master core owns pin  CPRD13=Master core owns pin  CPRD14=Master core owns pin  CPRD15=Master core owns pin  CPRE0=Master core owns pin  CPRE1=Master core owns pin  CPRE2=Master core owns pin  CPRE3=Master core owns pin  CPRE4=Master core owns pin  CPRE5=Master core owns pin  CPRE6=Master core owns pin  CPRE7=Master core owns pin  CPRE8=Master core owns pin  CPRE9=Master core owns pin  CPRE10=Master core owns pin  CPRE11=Master core owns pin  CPRE12=Master core owns pin  CPRE13=Master core owns pin  CPRE14=Master core owns pin  CPRE15=Master core owns pin  S1FNOSC=Internal Fast RC (FRC) Oscillator with postscaler  S1IESO=Start up with FRC; then switch  S1OSCIOFNC=OSC2 is clock output  S1FCKSM=Both Clock switching and Fail-safe Clock Monitor are disabled  S1PLLKEN=S1PLLKEN_ON  S1RWDTPS=1:1048576  S1RCLKSEL=Always use LPRC  S1WINDIS=Watchdog Timer operates in Non-Window mode  S1WDTWIN=WDT Window is 25% of WDT period  S1SWDTPS=1:1048576  S1FWDTEN=use WDTCON.ON bit  S1ICS=Communicate on PGC1 and PGD1  S1DEBUG=Not used  S1ISOLAT=The slave can operate (in debug mode) even if the SLVEN bit in the MSI is zero  S1NOBTSWP=BOOTSWP instruction is disabled  S1ALTI2C1=I2C1 mapped to SDA1/SCL1 pins  S1SPI1PIN=Slave SPI1 uses I/O remap (PPS) pins  S1SSRE=Slave generated resets will reset the Slave Enable Bit in the MSI module  S1MSRE=The master software oriented RESET events (RESET Op-Code; Watchdog timeout; TRAP reset; illegalInstruction) will also cause the slave subsystem to reset  S1CTXT1=Not Assigned  S1CTXT2=Not Assigned  S1CTXT3=Not Assigned  S1CTXT4=Not Assigned  BORLVL=Not used  BSSO=Not used  MCA=Not used  MAXTEMP=Not used  CFGAN14=Not used  CFGAN15=Not used  S1IOL1WAY=Not used  S1BSSO=Not used  S1BACKBUG=Not used  BISTDIS=mBIST on reset feature disabled  NOBTSWP=BOOTSWP instruction is disabled  S1BISTDIS=Slave BIST on reset feature disabled  S1DMTIVTL=Not used  S1DMTIVTH=Not used  S1DMTCNTL=Not used  S1DMTCNTH=Not used  S1DMTDIS=Slave Dead Man Timer is Disabled and can be enabled by software  BSEQ=Not used  IBSEQ=Not used  SMB3EN=SMBus 3.0 input levels  FUSBIDIO2=USBID pin is controlled by the USB2 module  FVBUSIO2=VBUSON pin is controlled by the USB2 module  FUSBIDIO1=USBID pin is controlled by the USB1 module  FVBUSIO1=VBUSON pin is controlled by the USB1 module  VBATBOREN=Enable ZPBOR during VBAT Mode  FDSEN=Enable DSEN bit in DSCON  BORSEL=BOR trip voltage 2.1v (Non-OPAMP deviced operation)  POSCFGAIN=Gain is G3  POSCAGCDLY=Settling time = 25ms x AGCRNG  POSCAGCRNG=Range 1x  POSCAGC=Automatic Gain Control for Oscillator  FDBGWP=Not used
      settings: SourceProductName=MPLAB Device Blocks for Simulink
  Open board doc WWW : Subsystem
      settings: OpenFcn=web('https://www.microchip.com/dspic33ckcuriosity','-browser');
      mask Display: disp('Microstick Plus\nDev Board');
  PIL Profiling : MCHP_Blockset/Profiling/PIL Profiling  TIMER_Ressource=Dynamic Options  TIMER_Ressource_TXT=No constraints [Prefered]  TIMER_Ressource_Custom=[1]  TIMER_Resolution=Dynamic Options  TIMER_Resolution_TXT="Resol: 0.01111(us)  -  MaxPer: 0.728(ms)"  MCHP_TIMER_REQUEST={TIMER for PIL}{TmrCfg}20:1:1:0:[]:65536;  MCHP_TIMER_RESULT=[1 65535 ]  MCHP_MASTERLINK=dsPIC33CK_Curiosity_CRL_ExternalMode/Curiosity - dsPIC33CK256MP508/Microchip Master  Info="Timer 1:  Resol: 11.11111111(ns)  -  Max value: 728.167(us)"
      settings: SourceProductName=MPLAB Device Blocks for Simulink
  Port Info : MCHP_Blockset/System Info/Port Info  MCHP_MASTERLINK=dsPIC33CK_Curiosity_CRL_ExternalMode/Curiosity - dsPIC33CK256MP508/Microchip Master
      settings: SourceProductName=MPLAB Device Blocks for Simulink
  Timer Info : MCHP_Blockset/System Info/Timer Info  MCHP_MASTERLINK=dsPIC33CK_Curiosity_CRL_ExternalMode/Curiosity - dsPIC33CK256MP508/Microchip Master
      settings: SourceProductName=MPLAB Device Blocks for Simulink
  UART Configuration over USB : MCHP_Blockset/BUS UART/UART Configuration  UART_REF=3  BAUD_Choice=Dynamic Options  BAUD_Choice_TXT="460800         [-0.10%]"  BAUD_Choice_IR=Dynamic Options  BAUD_Choice_IR_TXT=[]  BAUD_Custom=115200  INT_PRIORITY=0  ALT_IO=on  PIN_RX=Dynamic Options  PIN_RX_TXT=D3 / P67 / Pin[69]  PIN_TX=Dynamic Options  PIN_TX_TXT=D4 / P68 / Pin[68]  MCHP_PORT="{UART3  Rx}{U3RX}3:0:P67;{UART3  Tx}{U3TX}3:1:P68;"  MCHP_MASTERLINK=dsPIC33CK_Curiosity_CRL_ExternalMode/Curiosity - dsPIC33CK256MP508/Microchip Master  MCHP_COM_ExtPil=on  TX_IMPLEMENTATION=Circular Buffer  TX_IMPLEMENTATION_default=Circular Buffer  TX_INT_PRIORITY=5  TX_INT_WHEN=is empty  TX_INT_WHEN_default=is empty & last char is sent  TX_CIRCULAR_SIZE=128  TX_DMA_CHANNEL="0   (Lowest Priority)"  TX_DMA_SIZE=[]  TX_TASK_PROTECTION=Delay tasks (default)  TX_INTERRUPT_PROTECTION=Do not send on conflict (default)  TX_INTERRUPT_PROTECTION_default=Do not send on conflict (default)  RX_IMPLEMENTATION=Circular Buffer  RX_IMPLEMENTATION_default=Circular Buffer  RX_INT_PRIORITY=6  RX_INT_WHEN=is 3/4 fulll (contains 3 data characters)  RX_CIRCULAR_SIZE=256  RX_DMA_CHANNEL=0  RX_DMA_SIZE=0  DuplexMode=Full duplex (default)  PIN_RX_Inv=off  PIN_TX_Inv=off  PIN_RXTX_Inv=off  ParityBit=No parity (default)  StopBit=1 stop bit (default)  IRDA=off  FlowControl=None  PIN_CTS=Dynamic Options  PIN_CTS_TXT=B0 / P32 / Pin[34]  PIN_RTS=Dynamic Options  PIN_RTS_TXT=B0 / P32 / Pin[34]  InitSequence_chkbox=off  BAUD_Choice_InitSeq=Dynamic Options  BAUD_Choice_InitSeq_TXT="115200         [-0.03%]"  BAUD_Choice_IR_InitSeq=Dynamic Options  BAUD_Choice_IR_InitSeq_TXT=0  BAUD_Custom_InitSeq=0  InitSequence='Hello World'
      settings: SourceProductName=MPLAB Device Blocks for Simulink
  wires:
  1Hz Blinking/1(Out1) -> Digital Output Write/1, Digital Output Write/4, Digital Output Write/3, Digital Output Write/2

== system dsPIC33CK_Curiosity_CRL_ExternalMode/Sin ==
  In1 : Inport
  Sin Double - Reference : Subsystem
  Sin Q15 : Subsystem
  Out1 : Outport  VectorParamsAs1DForOutWhenUnconnected=off
  Out2 : Outport  Port=2  VectorParamsAs1DForOutWhenUnconnected=off
  wires:
  In1/1 -> Sin Q15/1(In2), Sin Double - Reference/1(In1)
  Sin Q15/1(Sin_Out1) -> Out1/1
  Sin Double - Reference/1(Out1) -> Out2/1
  [Validation] -> Sin Double - Reference/Enable

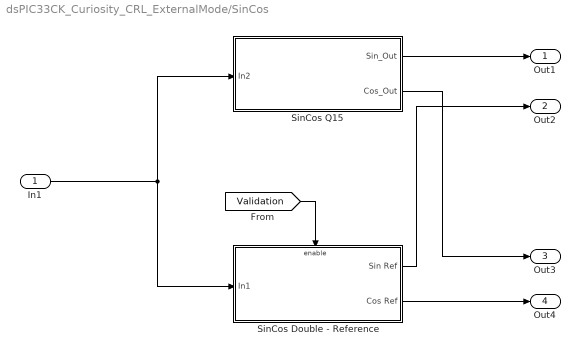
== system dsPIC33CK_Curiosity_CRL_ExternalMode/SinCos ==
  In1 : Inport
  SinCos Double - Reference : Subsystem
  SinCos Q15 : Subsystem
  Out1 : Outport  VectorParamsAs1DForOutWhenUnconnected=off
  Out2 : Outport  Port=2  VectorParamsAs1DForOutWhenUnconnected=off
  Out3 : Outport  Port=3  VectorParamsAs1DForOutWhenUnconnected=off
  Out4 : Outport  Port=4  VectorParamsAs1DForOutWhenUnconnected=off
  wires:
  In1/1 -> SinCos Q15/1(In2), SinCos Double - Reference/1(In1)
  SinCos Double - Reference/1(Sin Ref) -> Out2/1
  SinCos Double - Reference/2(Cos Ref) -> Out4/1
  SinCos Q15/2(Cos_Out) -> Out3/1
  SinCos Q15/1(Sin_Out) -> Out1/1
  [Validation] -> SinCos Double - Reference/Enable

== system dsPIC33CK_Curiosity_CRL_ExternalMode/Sqrt ==
  In1 : Inport
  " Sqrt Q15" : Subsystem  TreatAsAtomicUnit=on
  "Sqrt Double - Reference " : Subsystem  TreatAsAtomicUnit=on
  Out1 : Outport  VectorParamsAs1DForOutWhenUnconnected=off
  Out2 : Outport  Port=2  VectorParamsAs1DForOutWhenUnconnected=off
  wires:
  In1/1 -> " Sqrt Q15"/1(In1), "Sqrt Double - Reference "/1(In1)
  " Sqrt Q15"/1(Out1) -> Out1/1
  "Sqrt Double - Reference "/1(Out2) -> Out2/1
  [Validation] -> "Sqrt Double - Reference "/Enable

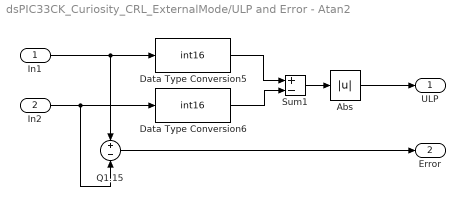
== system dsPIC33CK_Curiosity_CRL_ExternalMode/ULP and Error - Atan2 ==
  In1 : Inport
  In2 : Inport  Port=2
  Abs : Abs  SaturateOnIntegerOverflow=on
  Data Type Conversion5 : DataTypeConversion  OutDataTypeStr=int16  ConvertRealWorld=Stored Integer (SI)
  Data Type Conversion6 : DataTypeConversion  OutDataTypeStr=int16  ConvertRealWorld=Stored Integer (SI)
  Q1.15 : Sum  Inputs=+-  OutDataTypeStr=single
  Sum1 : Sum  Inputs=+-  SaturateOnIntegerOverflow=on  OutDataTypeStr=Inherit: Same as first input
  ULP : Outport  VectorParamsAs1DForOutWhenUnconnected=off
  Error : Outport  Port=2  VectorParamsAs1DForOutWhenUnconnected=off
  wires:
  Abs/1 -> ULP/1
  Q1.15/1 -> Error/1
  In1/1 -> Q1.15/1, Data Type Conversion5/1
  In2/1 -> Data Type Conversion6/1, Q1.15/2
  Sum1/1 -> Abs/1
  Data Type Conversion5/1 -> Sum1/1
  Data Type Conversion6/1 -> Sum1/2

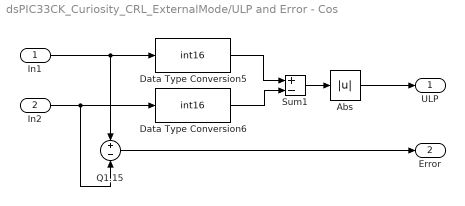
== system dsPIC33CK_Curiosity_CRL_ExternalMode/ULP and Error - Cos ==
  In1 : Inport
  In2 : Inport  Port=2
  Abs : Abs  SaturateOnIntegerOverflow=on
  Data Type Conversion5 : DataTypeConversion  OutDataTypeStr=int16  ConvertRealWorld=Stored Integer (SI)
  Data Type Conversion6 : DataTypeConversion  OutDataTypeStr=int16  ConvertRealWorld=Stored Integer (SI)
  Q1.15 : Sum  Inputs=+-  OutDataTypeStr=single
  Sum1 : Sum  Inputs=+-  SaturateOnIntegerOverflow=on  OutDataTypeStr=Inherit: Same as first input
  ULP : Outport  VectorParamsAs1DForOutWhenUnconnected=off
  Error : Outport  Port=2  VectorParamsAs1DForOutWhenUnconnected=off
  wires:
  Abs/1 -> ULP/1
  Q1.15/1 -> Error/1
  In1/1 -> Q1.15/1, Data Type Conversion5/1
  In2/1 -> Data Type Conversion6/1, Q1.15/2
  Sum1/1 -> Abs/1
  Data Type Conversion5/1 -> Sum1/1
  Data Type Conversion6/1 -> Sum1/2

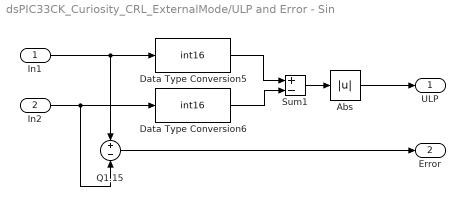
== system dsPIC33CK_Curiosity_CRL_ExternalMode/ULP and Error - Sin ==
  In1 : Inport
  In2 : Inport  Port=2
  Abs : Abs  SaturateOnIntegerOverflow=on
  Data Type Conversion5 : DataTypeConversion  OutDataTypeStr=int16  ConvertRealWorld=Stored Integer (SI)
  Data Type Conversion6 : DataTypeConversion  OutDataTypeStr=int16  ConvertRealWorld=Stored Integer (SI)
  Q1.15 : Sum  Inputs=+-  OutDataTypeStr=single
  Sum1 : Sum  Inputs=+-  SaturateOnIntegerOverflow=on  OutDataTypeStr=Inherit: Same as first input
  ULP : Outport  VectorParamsAs1DForOutWhenUnconnected=off
  Error : Outport  Port=2  VectorParamsAs1DForOutWhenUnconnected=off
  wires:
  Data Type Conversion6/1 -> Sum1/2
  Data Type Conversion5/1 -> Sum1/1
  Sum1/1 -> Abs/1
  In2/1 -> Q1.15/2, Data Type Conversion6/1
  In1/1 -> Data Type Conversion5/1, Q1.15/1
  Q1.15/1 -> Error/1
  Abs/1 -> ULP/1
